simulink model "testFurnace"  (R2025a)
settings: Solver=VariableStepAuto  StartTime=0.0  StopTime=10.0  RelTol=1e-3
libraries: StdLib x11, ProductionLinePLib x1
settings Model: Creator=peter  LastModifiedBy=peter
settings RTWCC: GPUComputeCapability=3.5

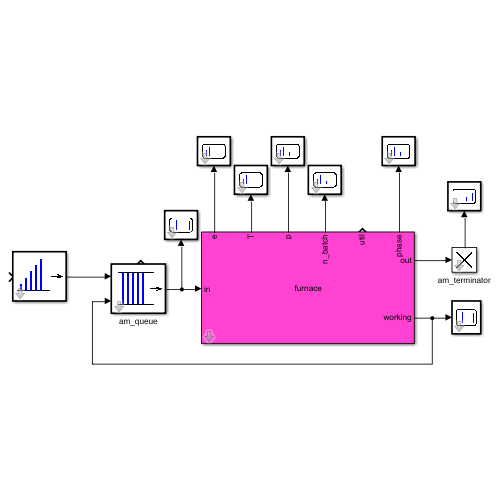
[thumbnail: Simulink's stored preview of the top-level diagram]
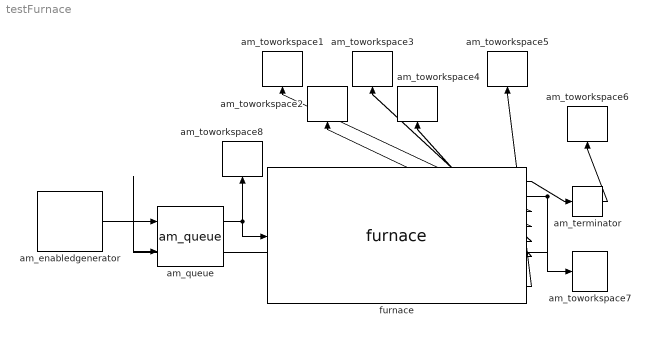
== system testFurnace ==
  am_enabledgenerator : StdLib/am_enabledgenerator  tG=500  n0=1  nG=80  tD=[0,2]  tau=[0,1]  debug=0
  am_queue : StdLib/am_queue  tD=[0,5]  tau=[0,5]  debug=0
  am_terminator : StdLib/am_terminator  tau=[0,1]  debug=0
  am_toworkspace1 : StdLib/am_toworkspace  varname="\"E\""  t0=0  format="\"vector\""  tau=[0,5]  debug=0
  am_toworkspace2 : StdLib/am_toworkspace  varname="\"T\""  t0=0  format="\"vector\""  tau=[0,5]  debug=0
  am_toworkspace3 : StdLib/am_toworkspace  varname="\"P\""  t0=0  format="\"vector\""  tau=[0,5]  debug=0
  am_toworkspace4 : StdLib/am_toworkspace  varname="\"batch\""  t0=0  format="\"vector\""  tau=[0,5]  debug=0
  am_toworkspace5 : StdLib/am_toworkspace  varname="\"phase\""  t0=0  format="\"vector\""  tau=[0,5]  debug=0
  am_toworkspace6 : StdLib/am_toworkspace  varname="\"Term_n\""  t0=0  format="\"vector\""  tau=[0,5]  debug=0
  am_toworkspace7 : StdLib/am_toworkspace  varname="\"working\""  t0=0  format="\"vector\""  tau=[0,5]  debug=0
  am_toworkspace8 : StdLib/am_toworkspace  varname="\"FIFO_n\""  t0=0  format="\"vector\""  tau=[0,1]  debug=0
  furnace : ProductionLinePLib/furnace  PH=6400  Co=6000  k_A=6  Te=25  P0=2000  P_unload=60000  holding_time=5400  Tsoll=800  Kapa=20  tauInt=[0,100]  tauCont=[0,100]  tau=[0,1]  debug=0
  wires:
  am_enabledgenerator/1 -> am_queue/1
  am_queue/1 -> am_toworkspace8/1, furnace/1
  furnace/1 -> am_terminator/1
  furnace/2 -> am_toworkspace7/1, am_queue/2
  furnace/4 -> am_toworkspace2/1
  furnace/5 -> am_toworkspace3/1
  furnace/3 -> am_toworkspace1/1
  am_terminator/1 -> am_toworkspace6/1
  furnace/6 -> am_toworkspace4/1
  furnace/8 -> am_toworkspace5/1
